simulink model "System_20220515"  (R2020b)
settings: Solver=ode4  StartTime=0.0  StopTime=inf  FixedStep=Ts  RelTol=1e-3  EnableMultiTasking=on
PreLoadFcn:
  | simulation_vars
PostLoadFcn:
  | simulation_vars
InitFcn:
  | simulation_vars
StartFcn:
  | simulation_vars
values from neighbouring files (symbols this model uses):
  ang_variance = 0.001*60    (= 0.06)    [simulation_vars.m]
  bus_va_seed = abs(round(1000*randn(73,1)))    [simulation_vars.m]
  bus_vm_seed = abs(round(1000*randn(73,1)))    [simulation_vars.m]
  event_time_end = event_time_start + 5/60    (= 10000.0833333)    [simulation_vars.m]
  event_time_start = 10000    [simulation_vars.m]
  line_iang0_seed = abs(round(1000*randn(104,1)))    [simulation_vars.m]
  line_iang1_seed = abs(round(1000*randn(104,1)))    [simulation_vars.m]
  line_imag0_seed = abs(round(1000*randn(104,1)))    [simulation_vars.m]
  line_imag1_seed = abs(round(1000*randn(104,1)))    [simulation_vars.m]
  mag_variance = 0.0005    [simulation_vars.m]
  spoof_lower_limit = -pi()/9    [simulation_vars.m]
  spoof_upper_limit = pi()/9    [simulation_vars.m]
  Ts = 0.001    [simulation_vars.m]
  xf_iang0_seed = abs(round(1000*randn(16,1)))    [simulation_vars.m]
  xf_iang1_seed = abs(round(1000*randn(16,1)))    [simulation_vars.m]
  xf_imag0_seed = abs(round(1000*randn(16,1)))    [simulation_vars.m]
  xf_imag1_seed = abs(round(1000*randn(16,1)))    [simulation_vars.m]
undefined symbols (not defined in the file or in its folder): en_spoofing_attack
libraries: rtlab x210, simulink x21, opal_lib x1, rtlab_phasor x1, rtio_spectracom x1
(part 4 of 4)

== system System_20220515/sm_master/PMU207_signals/Spoofing attack ==
  note: Modify demux and mux to fit input size.
      | Only modifies the angle measurements.
  Input : Inport
  Add : Sum
  Constant : Constant  Value=en_spoofing_attack.pmu_207
  Demux : Demux
  Demux1 : Demux  Outputs=2
  Multiply : Product
  Mux : Mux
  Mux1 : Mux  Inputs=2
  Ramp : simulink/Sources/Ramp  slope=1*pi()/180  start=spoof_st.pmu_207  InitialOutput=0
  Saturation : Saturate  UpperLimit=spoof_upper_limit  LowerLimit=spoof_lower_limit
  Output : Outport  VectorParamsAs1DForOutWhenUnconnected=off
  wires:
  Multiply/1 -> Add/1
  Saturation/1 -> Multiply/1
  Constant/1 -> Multiply/2
  Ramp/1 -> Saturation/1
  Input/1 -> Demux/1
  Mux/1 -> Output/1
  Demux/1 -> Mux/1
  Demux/3 -> Mux/3
  Demux/4 -> Mux1/2
  Demux/2 -> Mux1/1
  Mux1/1 -> Add/2
  Add/1 -> Demux1/1
  Demux1/1 -> Mux/2
  Demux1/2 -> Mux/4

== system System_20220515/sm_master/PMU210_signals/Spoofing attack ==
  note: Modify demux and mux to fit input size.
      | Only modifies the angle measurements.
  Input : Inport
  Add : Sum
  Constant : Constant  Value=en_spoofing_attack.pmu_210
  Demux : Demux  Outputs=12
  Demux1 : Demux  Outputs=6
  Multiply : Product
  Mux : Mux  Inputs=12
  Mux1 : Mux  Inputs=6
  Ramp : simulink/Sources/Ramp  slope=1*pi()/180  start=spoof_st.pmu_210  InitialOutput=0
  Saturation : Saturate  UpperLimit=spoof_upper_limit  LowerLimit=spoof_lower_limit
  Output : Outport  VectorParamsAs1DForOutWhenUnconnected=off
  wires:
  Multiply/1 -> Add/1
  Saturation/1 -> Multiply/1
  Constant/1 -> Multiply/2
  Ramp/1 -> Saturation/1
  Input/1 -> Demux/1
  Mux/1 -> Output/1
  Demux/1 -> Mux/1
  Demux/3 -> Mux/3
  Demux/5 -> Mux/5
  Demux/7 -> Mux/7
  Demux/9 -> Mux/9
  Demux/10 -> Mux1/5
  Demux/8 -> Mux1/4
  Demux/6 -> Mux1/3
  Demux/4 -> Mux1/2
  Demux/2 -> Mux1/1
  Mux1/1 -> Add/2
  Add/1 -> Demux1/1
  Demux1/1 -> Mux/2
  Demux1/2 -> Mux/4
  Demux1/3 -> Mux/6
  Demux1/4 -> Mux/8
  Demux1/5 -> Mux/10
  Demux/11 -> Mux/11
  Demux/12 -> Mux1/6
  Demux1/6 -> Mux/12

== system System_20220515/sm_master/PMU216_signals/Spoofing attack ==
  note: Modify demux and mux to fit input size.
      | Only modifies the angle measurements.
  Input : Inport
  Add : Sum
  Constant : Constant  Value=en_spoofing_attack.pmu_216
  Demux : Demux  Outputs=10
  Demux1 : Demux  Outputs=5
  Multiply : Product
  Mux : Mux  Inputs=10
  Mux1 : Mux  Inputs=5
  Ramp : simulink/Sources/Ramp  slope=1*pi()/180  start=spoof_st.pmu_216  InitialOutput=0
  Saturation : Saturate  UpperLimit=spoof_upper_limit  LowerLimit=spoof_lower_limit
  Output : Outport  VectorParamsAs1DForOutWhenUnconnected=off
  wires:
  Multiply/1 -> Add/1
  Saturation/1 -> Multiply/1
  Constant/1 -> Multiply/2
  Ramp/1 -> Saturation/1
  Input/1 -> Demux/1
  Mux/1 -> Output/1
  Demux/1 -> Mux/1
  Demux/3 -> Mux/3
  Demux/5 -> Mux/5
  Demux/7 -> Mux/7
  Demux/9 -> Mux/9
  Demux/10 -> Mux1/5
  Demux/8 -> Mux1/4
  Demux/6 -> Mux1/3
  Demux/4 -> Mux1/2
  Demux/2 -> Mux1/1
  Mux1/1 -> Add/2
  Add/1 -> Demux1/1
  Demux1/1 -> Mux/2
  Demux1/2 -> Mux/4
  Demux1/3 -> Mux/6
  Demux1/4 -> Mux/8
  Demux1/5 -> Mux/10

== system System_20220515/sm_master/PMU221_signals/Spoofing attack ==
  note: Modify demux and mux to fit input size.
      | Only modifies the angle measurements.
  Input : Inport
  Add : Sum
  Constant : Constant  Value=en_spoofing_attack.pmu_221
  Demux : Demux  Outputs=12
  Demux1 : Demux  Outputs=6
  Multiply : Product
  Mux : Mux  Inputs=12
  Mux1 : Mux  Inputs=6
  Ramp : simulink/Sources/Ramp  slope=1*pi()/180  start=spoof_st.pmu_221  InitialOutput=0
  Saturation : Saturate  UpperLimit=spoof_upper_limit  LowerLimit=spoof_lower_limit
  Output : Outport  VectorParamsAs1DForOutWhenUnconnected=off
  wires:
  Multiply/1 -> Add/1
  Saturation/1 -> Multiply/1
  Constant/1 -> Multiply/2
  Ramp/1 -> Saturation/1
  Input/1 -> Demux/1
  Mux/1 -> Output/1
  Demux/1 -> Mux/1
  Demux/3 -> Mux/3
  Demux/5 -> Mux/5
  Demux/7 -> Mux/7
  Demux/9 -> Mux/9
  Demux/10 -> Mux1/5
  Demux/8 -> Mux1/4
  Demux/6 -> Mux1/3
  Demux/4 -> Mux1/2
  Demux/2 -> Mux1/1
  Mux1/1 -> Add/2
  Add/1 -> Demux1/1
  Demux1/1 -> Mux/2
  Demux1/2 -> Mux/4
  Demux1/3 -> Mux/6
  Demux1/4 -> Mux/8
  Demux1/5 -> Mux/10
  Demux/11 -> Mux/11
  Demux/12 -> Mux1/6
  Demux1/6 -> Mux/12

== system System_20220515/sm_master/PMU223_signals/Spoofing attack ==
  note: Modify demux and mux to fit input size.
      | Only modifies the angle measurements.
  Input : Inport
  Add : Sum
  Constant : Constant  Value=en_spoofing_attack.pmu_223
  Demux : Demux  Outputs=12
  Demux1 : Demux  Outputs=6
  Multiply : Product
  Mux : Mux  Inputs=12
  Mux1 : Mux  Inputs=6
  Ramp : simulink/Sources/Ramp  slope=1*pi()/180  start=spoof_st.pmu_223  InitialOutput=0
  Saturation : Saturate  UpperLimit=spoof_upper_limit  LowerLimit=spoof_lower_limit
  Output : Outport  VectorParamsAs1DForOutWhenUnconnected=off
  wires:
  Multiply/1 -> Add/1
  Saturation/1 -> Multiply/1
  Constant/1 -> Multiply/2
  Ramp/1 -> Saturation/1
  Input/1 -> Demux/1
  Mux/1 -> Output/1
  Demux/1 -> Mux/1
  Demux/3 -> Mux/3
  Demux/5 -> Mux/5
  Demux/7 -> Mux/7
  Demux/9 -> Mux/9
  Demux/10 -> Mux1/5
  Demux/8 -> Mux1/4
  Demux/6 -> Mux1/3
  Demux/4 -> Mux1/2
  Demux/2 -> Mux1/1
  Mux1/1 -> Add/2
  Add/1 -> Demux1/1
  Demux1/1 -> Mux/2
  Demux1/2 -> Mux/4
  Demux1/3 -> Mux/6
  Demux1/4 -> Mux/8
  Demux1/5 -> Mux/10
  Demux/11 -> Mux/11
  Demux/12 -> Mux1/6
  Demux1/6 -> Mux/12

== system System_20220515/sm_master/PMU302_signals/Spoofing attack ==
  note: Modify demux and mux to fit input size.
      | Only modifies the angle measurements.
  Input : Inport
  Add : Sum
  Constant : Constant  Value=en_spoofing_attack.pmu_302
  Demux : Demux  Outputs=8
  Demux1 : Demux
  Multiply : Product
  Mux : Mux  Inputs=8
  Mux1 : Mux
  Ramp : simulink/Sources/Ramp  slope=1*pi()/180  start=spoof_st.pmu_302  InitialOutput=0
  Saturation : Saturate  UpperLimit=spoof_upper_limit  LowerLimit=spoof_lower_limit
  Output : Outport  VectorParamsAs1DForOutWhenUnconnected=off
  wires:
  Multiply/1 -> Add/1
  Saturation/1 -> Multiply/1
  Constant/1 -> Multiply/2
  Ramp/1 -> Saturation/1
  Input/1 -> Demux/1
  Mux/1 -> Output/1
  Demux/1 -> Mux/1
  Demux/3 -> Mux/3
  Demux/5 -> Mux/5
  Demux/7 -> Mux/7
  Demux/8 -> Mux1/4
  Demux/6 -> Mux1/3
  Demux/4 -> Mux1/2
  Demux/2 -> Mux1/1
  Mux1/1 -> Add/2
  Add/1 -> Demux1/1
  Demux1/1 -> Mux/2
  Demux1/2 -> Mux/4
  Demux1/3 -> Mux/6
  Demux1/4 -> Mux/8

== system System_20220515/sm_master/PMU303_signals/Spoofing attack ==
  note: Modify demux and mux to fit input size.
      | Only modifies the angle measurements.
  Input : Inport
  Add : Sum
  Constant : Constant  Value=en_spoofing_attack.pmu_303
  Demux : Demux  Outputs=8
  Demux1 : Demux
  Multiply : Product
  Mux : Mux  Inputs=8
  Mux1 : Mux
  Ramp : simulink/Sources/Ramp  slope=1*pi()/180  start=spoof_st.pmu_303  InitialOutput=0
  Saturation : Saturate  UpperLimit=spoof_upper_limit  LowerLimit=spoof_lower_limit
  Output : Outport  VectorParamsAs1DForOutWhenUnconnected=off
  wires:
  Multiply/1 -> Add/1
  Saturation/1 -> Multiply/1
  Constant/1 -> Multiply/2
  Ramp/1 -> Saturation/1
  Input/1 -> Demux/1
  Mux/1 -> Output/1
  Demux/1 -> Mux/1
  Demux/3 -> Mux/3
  Demux/5 -> Mux/5
  Demux/7 -> Mux/7
  Demux/8 -> Mux1/4
  Demux/6 -> Mux1/3
  Demux/4 -> Mux1/2
  Demux/2 -> Mux1/1
  Mux1/1 -> Add/2
  Add/1 -> Demux1/1
  Demux1/1 -> Mux/2
  Demux1/2 -> Mux/4
  Demux1/3 -> Mux/6
  Demux1/4 -> Mux/8

== system System_20220515/sm_master/PMU307_signals/Spoofing attack ==
  note: Modify demux and mux to fit input size.
      | Only modifies the angle measurements.
  Input : Inport
  Add : Sum
  Constant : Constant  Value=en_spoofing_attack.pmu_307
  Demux : Demux
  Demux1 : Demux  Outputs=2
  Multiply : Product
  Mux : Mux
  Mux1 : Mux  Inputs=2
  Ramp : simulink/Sources/Ramp  slope=1*pi()/180  start=spoof_st.pmu_307  InitialOutput=0
  Saturation : Saturate  UpperLimit=spoof_upper_limit  LowerLimit=spoof_lower_limit
  Output : Outport  VectorParamsAs1DForOutWhenUnconnected=off
  wires:
  Multiply/1 -> Add/1
  Saturation/1 -> Multiply/1
  Constant/1 -> Multiply/2
  Ramp/1 -> Saturation/1
  Input/1 -> Demux/1
  Mux/1 -> Output/1
  Demux/1 -> Mux/1
  Demux/3 -> Mux/3
  Demux/4 -> Mux1/2
  Demux/2 -> Mux1/1
  Mux1/1 -> Add/2
  Add/1 -> Demux1/1
  Demux1/1 -> Mux/2
  Demux1/2 -> Mux/4

== system System_20220515/sm_master/PMU310_signals/Spoofing attack ==
  note: Modify demux and mux to fit input size.
      | Only modifies the angle measurements.
  Input : Inport
  Add : Sum
  Constant : Constant  Value=en_spoofing_attack.pmu_310
  Demux : Demux  Outputs=12
  Demux1 : Demux  Outputs=6
  Multiply : Product
  Mux : Mux  Inputs=12
  Mux1 : Mux  Inputs=6
  Ramp : simulink/Sources/Ramp  slope=1*pi()/180  start=spoof_st.pmu_310  InitialOutput=0
  Saturation : Saturate  UpperLimit=spoof_upper_limit  LowerLimit=spoof_lower_limit
  Output : Outport  VectorParamsAs1DForOutWhenUnconnected=off
  wires:
  Multiply/1 -> Add/1
  Saturation/1 -> Multiply/1
  Constant/1 -> Multiply/2
  Ramp/1 -> Saturation/1
  Input/1 -> Demux/1
  Mux/1 -> Output/1
  Demux/1 -> Mux/1
  Demux/3 -> Mux/3
  Demux/5 -> Mux/5
  Demux/7 -> Mux/7
  Demux/9 -> Mux/9
  Demux/10 -> Mux1/5
  Demux/8 -> Mux1/4
  Demux/6 -> Mux1/3
  Demux/4 -> Mux1/2
  Demux/2 -> Mux1/1
  Mux1/1 -> Add/2
  Add/1 -> Demux1/1
  Demux1/1 -> Mux/2
  Demux1/2 -> Mux/4
  Demux1/3 -> Mux/6
  Demux1/4 -> Mux/8
  Demux1/5 -> Mux/10
  Demux/11 -> Mux/11
  Demux/12 -> Mux1/6
  Demux1/6 -> Mux/12

== system System_20220515/sm_master/PMU316_signals/Spoofing attack ==
  note: Modify demux and mux to fit input size.
      | Only modifies the angle measurements.
  Input : Inport
  Add : Sum
  Constant : Constant  Value=en_spoofing_attack.pmu_316
  Demux : Demux  Outputs=10
  Demux1 : Demux  Outputs=5
  Multiply : Product
  Mux : Mux  Inputs=10
  Mux1 : Mux  Inputs=5
  Ramp : simulink/Sources/Ramp  slope=1*pi()/180  start=spoof_st.pmu_316  InitialOutput=0
  Saturation : Saturate  UpperLimit=spoof_upper_limit  LowerLimit=spoof_lower_limit
  Output : Outport  VectorParamsAs1DForOutWhenUnconnected=off
  wires:
  Multiply/1 -> Add/1
  Saturation/1 -> Multiply/1
  Constant/1 -> Multiply/2
  Ramp/1 -> Saturation/1
  Input/1 -> Demux/1
  Mux/1 -> Output/1
  Demux/1 -> Mux/1
  Demux/3 -> Mux/3
  Demux/5 -> Mux/5
  Demux/7 -> Mux/7
  Demux/9 -> Mux/9
  Demux/10 -> Mux1/5
  Demux/8 -> Mux1/4
  Demux/6 -> Mux1/3
  Demux/4 -> Mux1/2
  Demux/2 -> Mux1/1
  Mux1/1 -> Add/2
  Add/1 -> Demux1/1
  Demux1/1 -> Mux/2
  Demux1/2 -> Mux/4
  Demux1/3 -> Mux/6
  Demux1/4 -> Mux/8
  Demux1/5 -> Mux/10

== system System_20220515/sm_master/PMU321_signals/Spoofing attack ==
  note: Modify demux and mux to fit input size.
      | Only modify the angle measurements.
  Input : Inport
  Add : Sum
  Constant : Constant  Value=en_spoofing_attack.pmu_321
  Demux : Demux  Outputs=12
  Demux1 : Demux  Outputs=6
  Multiply : Product
  Mux : Mux  Inputs=12
  Mux1 : Mux  Inputs=6
  Ramp : simulink/Sources/Ramp  slope=1*pi()/180  start=spoof_st.pmu_321  InitialOutput=0
  Saturation : Saturate  UpperLimit=spoof_upper_limit  LowerLimit=spoof_lower_limit
  Output : Outport  VectorParamsAs1DForOutWhenUnconnected=off
  wires:
  Multiply/1 -> Add/1
  Saturation/1 -> Multiply/1
  Constant/1 -> Multiply/2
  Ramp/1 -> Saturation/1
  Input/1 -> Demux/1
  Mux/1 -> Output/1
  Demux/1 -> Mux/1
  Demux/3 -> Mux/3
  Demux/5 -> Mux/5
  Demux/7 -> Mux/7
  Demux/9 -> Mux/9
  Demux/11 -> Mux/11
  Demux/12 -> Mux1/6
  Demux/10 -> Mux1/5
  Demux/8 -> Mux1/4
  Demux/6 -> Mux1/3
  Demux/4 -> Mux1/2
  Demux/2 -> Mux1/1
  Mux1/1 -> Add/2
  Add/1 -> Demux1/1
  Demux1/1 -> Mux/2
  Demux1/2 -> Mux/4
  Demux1/3 -> Mux/6
  Demux1/4 -> Mux/8
  Demux1/5 -> Mux/10
  Demux1/6 -> Mux/12

== system System_20220515/sm_master/PMU323_signals/Spoofing attack ==
  note: Modify demux and mux to fit input size.
      | Only modify the angle measurements.
  Input : Inport
  Add : Sum
  Constant : Constant  Value=en_spoofing_attack.pmu_323
  Demux : Demux  Outputs=12
  Demux1 : Demux  Outputs=6
  Multiply : Product
  Mux : Mux  Inputs=12
  Mux1 : Mux  Inputs=6
  Ramp : simulink/Sources/Ramp  slope=1*pi()/180  start=spoof_st.pmu_323  InitialOutput=0
  Saturation : Saturate  UpperLimit=spoof_upper_limit  LowerLimit=spoof_lower_limit
  Output : Outport  VectorParamsAs1DForOutWhenUnconnected=off
  wires:
  Multiply/1 -> Add/1
  Saturation/1 -> Multiply/1
  Constant/1 -> Multiply/2
  Ramp/1 -> Saturation/1
  Input/1 -> Demux/1
  Mux/1 -> Output/1
  Demux/1 -> Mux/1
  Demux/3 -> Mux/3
  Demux/5 -> Mux/5
  Demux/7 -> Mux/7
  Demux/9 -> Mux/9
  Demux/11 -> Mux/11
  Demux/12 -> Mux1/6
  Demux/10 -> Mux1/5
  Demux/8 -> Mux1/4
  Demux/6 -> Mux1/3
  Demux/4 -> Mux1/2
  Demux/2 -> Mux1/1
  Mux1/1 -> Add/2
  Add/1 -> Demux1/1
  Demux1/1 -> Mux/2
  Demux1/2 -> Mux/4
  Demux1/3 -> Mux/6
  Demux1/4 -> Mux/8
  Demux1/5 -> Mux/10
  Demux1/6 -> Mux/12

== matlab function System_20220515/sm_master/bus_va_noise/MATLAB Function ==
  data: u input; y output
function y = wrap_angle(u)

max_val = 180;
min_val = -179.99;

if u > max_val
    u = u - round(u/(2*max_val))*max_val*2;
end

if u < min_val
    u = u + round(abs(u)/(2*max_val))*max_val*2;
end

y = u;

== matlab function System_20220515/sm_master/line_iang1_noise/MATLAB Function ==
  data: u input; y output
function y = wrap_angle(u)

max_val = 180;
min_val = -179.99;

if u > max_val
    u = u - round(u/(2*max_val))*max_val*2;
end

if u < min_val
    u = u + round(abs(u)/(2*max_val))*max_val*2;
end

y = u;

== matlab function System_20220515/sm_master/xf_iang0_noise/MATLAB Function ==
  data: u input; y output
function y = wrap_angle(u)

max_val = 180;
min_val = -179.99;

if u > max_val
    u = u - round(u/(2*max_val))*max_val*2;
end

if u < min_val
    u = u + round(abs(u)/(2*max_val))*max_val*2;
end

y = u;

== matlab function System_20220515/sm_master/xf_iang1_noise/MATLAB Function ==
  data: u input; y output
function y = wrap_angle(u)

max_val = 180;
min_val = -179.99;

if u > max_val
    u = u - round(u/(2*max_val))*max_val*2;
end

if u < min_val
    u = u + round(abs(u)/(2*max_val))*max_val*2;
end

y = u;

== matlab function System_20220515/sm_master/line_iang0_noise/MATLAB Function ==
  data: u input; y output
function y = wrap_angle(u)

max_val = 180;
min_val = -179.99;

if u > max_val
    u = u - round(u/(2*max_val))*max_val*2;
end

if u < min_val
    u = u + round(abs(u)/(2*max_val))*max_val*2;
end

y = u;
